simulink model "model"  (Simulink 7.8)
settings: Solver=ode5  StartTime=0.0  StopTime=10.0  FixedStep=Ts  RelTol=1e-3
values from neighbouring files (symbols this model uses):
  g = 9.8065    [kostas_malakies.mat]    (also in kostas_malakies2.mat; load_PMModel.m = 9.81; main_last.m; matlab.mat)
  mass = 0.66    [kostas_malakies.mat]    (also in kostas_malakies2.mat; load_PMModel.m = 0.687; main_last.m)
  Ts = 0.02    [kostas_malakies.mat]    (also in kostas_malakies2.mat; main.m; main_last.m; matlab.mat = 0.08)
  yaw0 = 0    [kostas_malakies.mat]    (also in kostas_malakies2.mat; main.m; main_last.m; matlab.mat = -0.0873)
libraries: Hqaud_model_LIB_SI x5
settings Model: Creator=burrimi  LastModifiedBy=burrimi
settings DataIOCC: SaveOutput=off  SaveTime=off
settings OptimizationCC: ZeroExternalMemoryAtStartup=off  OptimizeModelRefInitCode=on  LifeSpan=1
settings DebuggingCC: FcnCallInpInsideContextMsg=Use local settings
settings HardwareCC: ProdIntDivRoundTo=Zero  ProdEndianess=LittleEndian  ProdHWDeviceType=Intel Pentium  TargetBitPerLong=64  TargetBitPerPointer=64  TargetIntDivRoundTo=Zero  TargetEndianess=LittleEndian  TargetWordSize=64  TargetHWDeviceType=MATLAB Host
settings RTWCC: SystemTargetFile=ert.tlc  TemplateMakefile=ert_default_tmf  Description=Real-Time Workshop Embedded Coder  GenerateReport=on  ProcessScript=ert_make_rtw_hook  IncludeHyperlinkInReport=on  LaunchReport=on  TargetLang=C++ (Encapsulated)
settings ERTTargetCC: MultiwordLength=2048  GenerateSampleERTMain=on  MultiInstanceERTCode=on  SupportContinuousTime=on  RootIOFormat=Structure reference  ERTCustomFileTemplate=example_file_process.tlc  ConvertIfToSwitch=off  SuppressUnreachableDefaultCases=off
settings ERTCPPComponent: GenerateDestructor=on  GenerateExternalIOAccessMethods=None  ParameterMemberVisibility=private  InternalMemberVisibility=private  GenerateParameterAccessMethods=None  GenerateInternalMemberAccessMethods=None  UseOperatorNewForModelRefRegistration=off

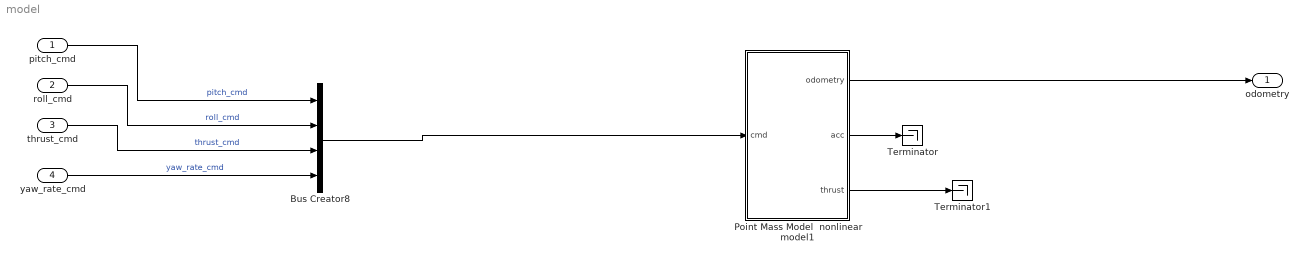
== system model ==
  pitch_cmd : Inport  PortDimensions=1  SampleTime=Ts
  roll_cmd : Inport  Port=2  PortDimensions=1  SampleTime=Ts
  thrust_cmd : Inport  Port=3  PortDimensions=1  SampleTime=Ts
  yaw_rate_cmd : Inport  Port=4  PortDimensions=1  SampleTime=Ts
  Bus Creator8 : BusCreator
  Point Mass Model  nonlinear model1 : Subsystem  AncestorBlock="Hqaud_model_LIB_SI/Point Mass Model  nonlinear model"
  Terminator : Terminator
  Terminator1 : Terminator
  odometry : Outport  SampleTime=Ts
  wires:
  Point Mass Model  nonlinear model1/3("thrust   ") -> Terminator1/1
  Point Mass Model  nonlinear model1/2(acc) -> Terminator/1
  Point Mass Model  nonlinear model1/1(odometry) -> odometry/1
  pitch_cmd/1 -> Bus Creator8/1  "pitch_cmd"
  roll_cmd/1 -> Bus Creator8/2  "roll_cmd"
  thrust_cmd/1 -> Bus Creator8/3  "thrust_cmd"
  yaw_rate_cmd/1 -> Bus Creator8/4  "yaw_rate_cmd"
  Bus Creator8/1 -> Point Mass Model  nonlinear model1/1(cmd)

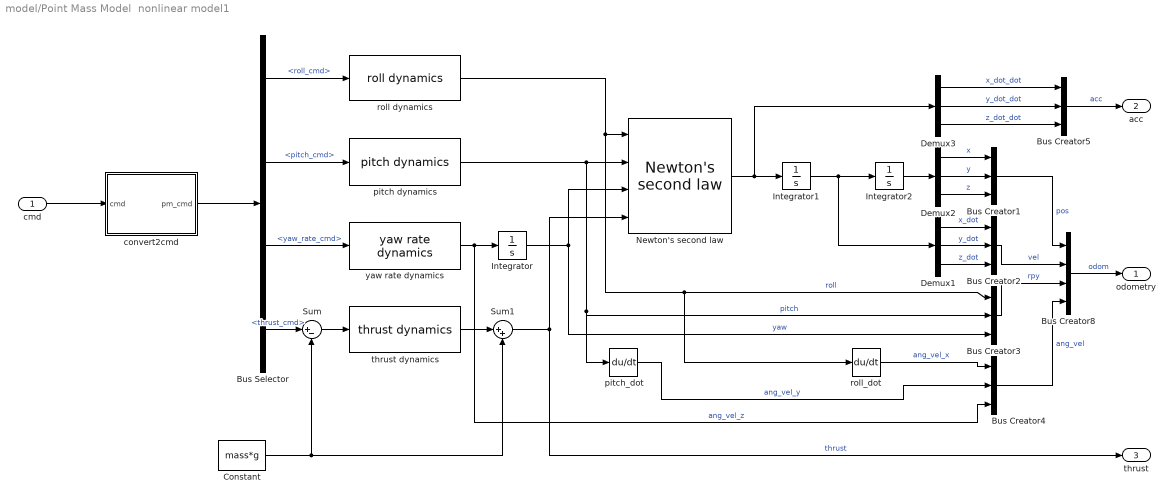
== system model/Point Mass Model  nonlinear model1 ==
  cmd : Inport
  Bus Creator{1..5} (5 alike) : BusCreator  Inputs=3
  Bus Creator8 : BusCreator
  Bus Selector : BusSelector  OutputSignals=roll_cmd,pitch_cmd,yaw_rate_cmd,thrust_cmd
  Constant : Constant  Value=mass*g
  Demux1 : Demux  Outputs=3
  Demux2 : Demux  Outputs=3
  Demux3 : Demux  Outputs=3
  Integrator : Integrator  InitialCondition=yaw0
  Integrator1 : Integrator
  Integrator2 : Integrator
  "Newton's second law  " : Hqaud_model_LIB_SI/Newton's second law  
  Sum : Sum  Inputs=|+-
  Sum1 : Sum  Inputs=|++
  convert2cmd : Subsystem
  "pitch dynamics  " : Hqaud_model_LIB_SI/pitch dynamics  
  pitch_dot : Derivative
  roll dynamics : Hqaud_model_LIB_SI/roll dynamics
  roll_dot : Derivative
  "thrust dynamics  " : Hqaud_model_LIB_SI/thrust dynamics  
  "yaw rate dynamics  " : Hqaud_model_LIB_SI/yaw rate dynamics  
  odometry : Outport
  acc : Outport  Port=2
  "thrust   " : Outport  Port=3  PortDimensions=1
  wires:
  convert2cmd/1(pm_cmd) -> Bus Selector/1
  Bus Selector/1 -> roll dynamics/1  "<roll_cmd>"
  "yaw rate dynamics  "/1 -> Integrator/1, Bus Creator4/3  "ang_vel_z"
  Integrator/1 -> "Newton's second law  "/3, Bus Creator3/3  "yaw"
  "thrust dynamics  "/1 -> Sum1/1
  "pitch dynamics  "/1 -> "Newton's second law  "/2, Bus Creator3/2, pitch_dot/1  "pitch"
  roll dynamics/1 -> "Newton's second law  "/1, Bus Creator3/1, roll_dot/1  "roll"
  "Newton's second law  "/1 -> Integrator1/1, Demux3/1
  Integrator1/1 -> Integrator2/1, Demux1/1
  Integrator2/1 -> Demux2/1
  Demux2/2 -> Bus Creator1/2  "y"
  Constant/1 -> Sum/2, Sum1/2
  Sum/1 -> "thrust dynamics  "/1
  Bus Selector/4 -> Sum/1  "<thrust_cmd>"
  cmd/1 -> convert2cmd/1(cmd)
  Bus Selector/2 -> "pitch dynamics  "/1  "<pitch_cmd>"
  Bus Selector/3 -> "yaw rate dynamics  "/1  "<yaw_rate_cmd>"
  Bus Creator4/1 -> Bus Creator8/4  "ang_vel"
  Bus Creator3/1 -> Bus Creator8/3  "rpy"
  Bus Creator2/1 -> Bus Creator8/2  "vel"
  Bus Creator1/1 -> Bus Creator8/1  "pos"
  Bus Creator8/1 -> odometry/1  "odom"
  Demux2/3 -> Bus Creator1/3  "z"
  Demux2/1 -> Bus Creator1/1  "x"
  Demux1/1 -> Bus Creator2/1  "x_dot"
  Demux1/2 -> Bus Creator2/2  "y_dot"
  Demux1/3 -> Bus Creator2/3  "z_dot"
  Bus Creator5/1 -> acc/1  "acc"
  Demux3/1 -> Bus Creator5/1  "x_dot_dot"
  Demux3/2 -> Bus Creator5/2  "y_dot_dot"
  Demux3/3 -> Bus Creator5/3  "z_dot_dot"
  Sum1/1 -> "Newton's second law  "/4, "thrust   "/1  "thrust"
  roll_dot/1 -> Bus Creator4/1  "ang_vel_x"
  pitch_dot/1 -> Bus Creator4/2  "ang_vel_y"

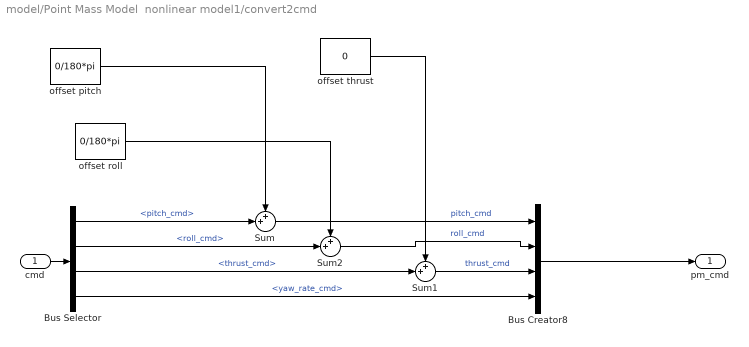
== system model/Point Mass Model  nonlinear model1/convert2cmd ==
  cmd : Inport
  Bus Creator8 : BusCreator
  Bus Selector : BusSelector  OutputSignals=pitch_cmd,roll_cmd,thrust_cmd,yaw_rate_cmd
  Sum : Sum  Inputs=++|
  Sum1 : Sum  Inputs=++|
  Sum2 : Sum  Inputs=++|
  offset pitch : Constant  Value=0/180*pi
  offset roll : Constant  Value=0/180*pi
  offset thrust : Constant  Value=0
  pm_cmd : Outport
  wires:
  Bus Selector/4 -> Bus Creator8/4  "<yaw_rate_cmd>"
  cmd/1 -> Bus Selector/1
  Bus Creator8/1 -> pm_cmd/1
  offset pitch/1 -> Sum/1
  Bus Selector/1 -> Sum/2  "<pitch_cmd>"
  Sum/1 -> Bus Creator8/1  "pitch_cmd"
  Bus Selector/3 -> Sum1/2  "<thrust_cmd>"
  Sum1/1 -> Bus Creator8/3  "thrust_cmd"
  offset thrust/1 -> Sum1/1
  Sum2/1 -> Bus Creator8/2  "roll_cmd"
  Bus Selector/2 -> Sum2/2  "<roll_cmd>"
  offset roll/1 -> Sum2/1
